simulink model "yaw_sim"  (R2021b)
settings: Solver=VariableStepAuto  StartTime=0.0  StopTime=20  RelTol=1e-3
values from neighbouring files (symbols this model uses):
  F_g = 0.63    [lab3_workspace.m]
  J_ps = 1.1    [lab3_workspace.m]
  K_r_i = 0.03*K_r_p    [lab3_workspace.m]
  K_r_p = (J_ps/(F_g*l_a*tau))*0.65    [lab3_workspace.m]
  l_a = 0.63    [lab3_workspace.m]
settings Model: Creator=DSDLn  LastModifiedBy=DSDLn

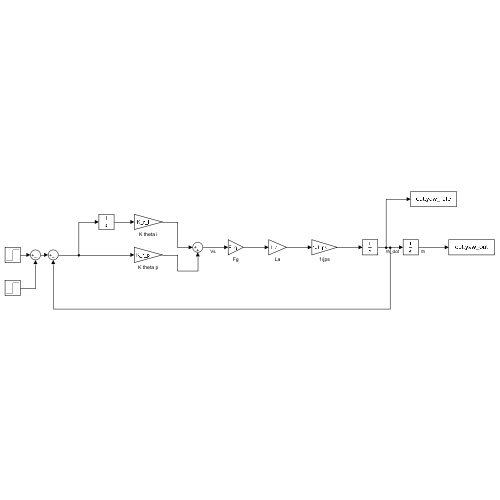
[thumbnail: Simulink's stored preview of the top-level diagram]
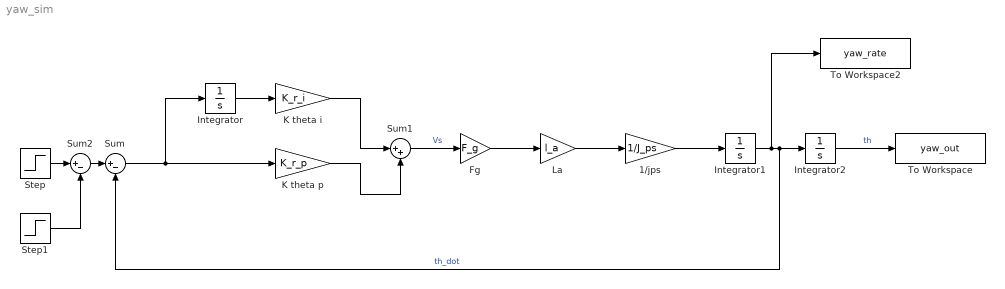
== system yaw_sim ==
  1/jps : Gain  Gain=1/J_ps
  Fg : Gain  Gain=F_g
  Integrator : Integrator
  Integrator1 : Integrator
  Integrator2 : Integrator
  K theta i : Gain  Gain=K_r_i
  K theta p : Gain  Gain=K_r_p
  La : Gain  Gain=l_a
  Step : Step  Time=0  After=deg2rad(10)  SampleTime=0.01
  Step1 : Step  Time=10  After=deg2rad(10)  SampleTime=0.01
  Sum : Sum  Inputs=|+-
  Sum1 : Sum  Inputs=|++
  Sum2 : Sum  Inputs=|+-
  To Workspace : ToWorkspace  VariableName=yaw_out  SampleTime=-1
  To Workspace2 : ToWorkspace  VariableName=yaw_rate  SampleTime=-1
  wires:
  K theta p/1 -> Sum1/2
  Sum1/1 -> Fg/1  "Vs"
  K theta i/1 -> Sum1/1
  Fg/1 -> La/1
  1/jps/1 -> Integrator1/1
  La/1 -> 1/jps/1
  Integrator1/1 -> Sum/2, Integrator2/1, To Workspace2/1  "th_dot"
  Integrator2/1 -> To Workspace/1  "th"
  Sum/1 -> K theta p/1, Integrator/1
  Integrator/1 -> K theta i/1
  Step/1 -> Sum2/1
  Sum2/1 -> Sum/1
  Step1/1 -> Sum2/2
